simulink model "DAB_Model"  (R2025a)
settings: Solver=VariableStepAuto  StartTime=0.0  StopTime=10.0  RelTol=1e-3
settings Model: Creator=hridoyshakil  LastModifiedBy=hridoyshakil

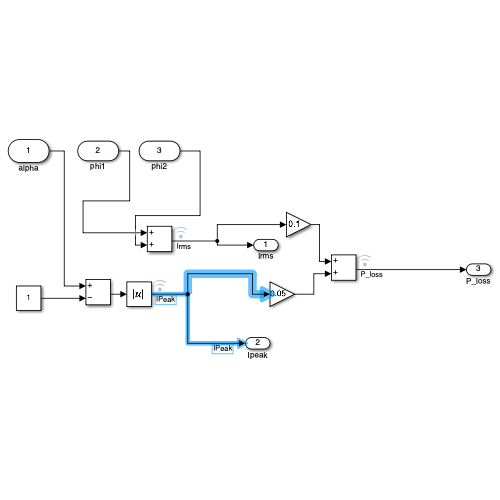
[thumbnail: Simulink's stored preview of the top-level diagram]
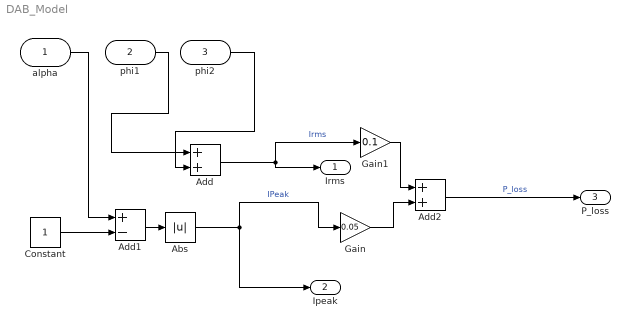
== system DAB_Model ==
  alpha : Inport
  phi1 : Inport  Port=2
  phi2 : Inport  Port=3
  Abs : Abs  SaturateOnIntegerOverflow=off
  Add : Sum
  Add1 : Sum  Inputs=+-
  Add2 : Sum
  Constant : Constant
  Gain : Gain  Gain=0.05
  Gain1 : Gain  Gain=0.1
  Irms : Outport
  Ipeak : Outport  Port=2
  P_loss : Outport  Port=3
  wires:
  phi1/1 -> Add/1
  phi2/1 -> Add/2
  alpha/1 -> Add1/1
  Constant/1 -> Add1/2
  Add1/1 -> Abs/1
  Abs/1 -> Ipeak/1, Gain/1  "IPeak"
  Gain/1 -> Add2/2
  Gain1/1 -> Add2/1
  Add2/1 -> P_loss/1  "P_loss"
  Add/1 -> Irms/1, Gain1/1  "Irms"
